simulink library "eng_simple_transient_std"  (Simulink 8.7)
settings: Solver=ode45  StartTime=0.0  StopTime=10.0  RelTol=1e-3
undefined symbols (not defined in the file): DiscIntNeverNeededParam, sMP
libraries: simulink x17
(part 2 of 3)

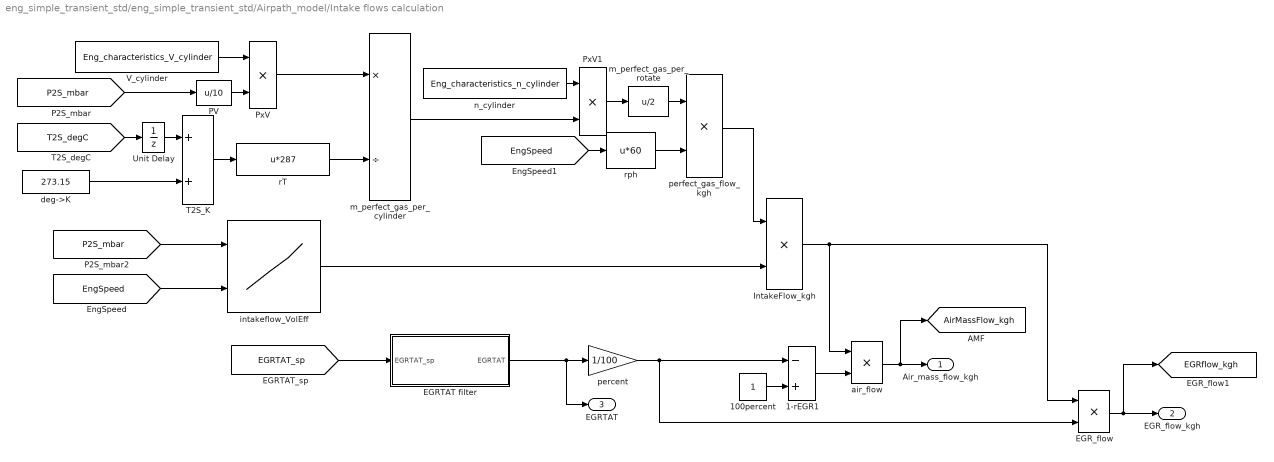
== system eng_simple_transient_std/eng_simple_transient_std/Airpath_model/Intake flows calculation ==
  1-rEGR1 : Sum  Inputs=-+
  100percent : Constant
  EGRTAT filter : Subsystem  AncestorBlock=ControlLib/# First order filter
  EGR_flow : Product  Inputs=**
  IntakeFlow_kgh : Product  RndMeth=Zero
  PV : Fcn  Expr=u/10
  PxV : Product  RndMeth=Zero
  PxV1 : Product  RndMeth=Zero
  T2S_K : Sum
  Unit Delay : UnitDelay  SampleTime=-1
  V_cylinder : Constant  Value=Eng_characteristics_V_cylinder
  air_flow : Product  Inputs=**
  deg->K : Constant  Value=273.15
  intakeflow_VolEff : Lookup2D  RowIndex=Airpath_intakeflow_y_P2S_mbar  ColumnIndex=Airpath_intakeflow_x_NMOTW_rpm  Table=Airpath_intakeflow_z_VolEff  LookUpMeth=Interpolation-Use End Values
  m_perfect_gas_per_cylinder : Product  Inputs=*/
  m_perfect_gas_per_rotate : Fcn  Expr=u/2
  n_cylinder : Constant  Value=Eng_characteristics_n_cylinder
  percent : Gain  Gain=1/100
  perfect_gas_flow_kgh : Product  RndMeth=Zero
  rT : Fcn  Expr=u*287
  rph : Fcn  Expr=u*60
  Air_mass_flow_kgh : Outport
  EGR_flow_kgh : Outport  Port=2
  EGRTAT : Outport  Port=3
  tag scope: AirMassFlow_kgh=global, EGRflow_kgh=global
  wires:
  PxV1/1 -> m_perfect_gas_per_rotate/1
  m_perfect_gas_per_cylinder/1 -> PxV1/2
  n_cylinder/1 -> PxV1/1
  PxV/1 -> m_perfect_gas_per_cylinder/1
  V_cylinder/1 -> PxV/1
  PV/1 -> PxV/2
  Unit Delay/1 -> T2S_K/1
  perfect_gas_flow_kgh/1 -> IntakeFlow_kgh/1
  rph/1 -> perfect_gas_flow_kgh/2
  m_perfect_gas_per_rotate/1 -> perfect_gas_flow_kgh/1
  [EngSpeed] -> rph/1
  [P2S_mbar] -> intakeflow_VolEff/1
  [EngSpeed] -> intakeflow_VolEff/2
  [P2S_mbar] -> PV/1
  deg->K/1 -> T2S_K/2
  [T2S_degC] -> Unit Delay/1
  rT/1 -> m_perfect_gas_per_cylinder/2
  T2S_K/1 -> rT/1
  intakeflow_VolEff/1 -> IntakeFlow_kgh/2
  IntakeFlow_kgh/1 -> air_flow/1, EGR_flow/1
  [EGRTAT_sp] -> EGRTAT filter/1(EGRTAT_sp)
  EGRTAT filter/1(EGRTAT) -> EGRTAT/1, percent/1
  100percent/1 -> 1-rEGR1/2
  percent/1 -> EGR_flow/2, 1-rEGR1/1
  1-rEGR1/1 -> air_flow/2
  EGR_flow/1 -> [EGRflow_kgh], EGR_flow_kgh/1
  air_flow/1 -> [AirMassFlow_kgh], Air_mass_flow_kgh/1

== system eng_simple_transient_std/eng_simple_transient_std/Engine_model/AFR calculation ==
  AFR calc : Product  Inputs=*//
  Saturation : Saturate  UpperLimit=20  LowerLimit=0
  Saturation1 : Saturate  UpperLimit=1e6  LowerLimit=1e-6
  Stoech_coeff : Constant  Value=Eng_characteristics_Stoech_coeff
  AFR : Outport
  wires:
  [MFuel_kgh] -> Saturation1/1
  Saturation1/1 -> AFR calc/2
  Saturation/1 -> AFR/1
  AFR calc/1 -> Saturation/1
  Stoech_coeff/1 -> AFR calc/3
  [AirMassFlow_kgh] -> AFR calc/1

== system eng_simple_transient_std/eng_simple_transient_std/Engine_model/AdBlue consumption ==
  Calc_AdBlue_Consumption : Subsystem
  Discrete-Time Integrator : DiscreteIntegrator  SampleTime=-1  ICPrevOutput=DiscIntNeverNeededParam  ICPrevScaledInput=DiscIntNeverNeededParam
  Divide : Product  Inputs=*/
  Divide1 : Product  Inputs=*/
  fuel_density : Constant  Value=Eng_characteristics_AdBlue_density
  kgh->kgs : Gain  Gain=1/3600
  MAdBlue_brk_kgh : Outport
  VAdBlue_Lh : Outport  Port=2
  MAdBlue_kg : Outport  Port=3
  VAdBlue_L : Outport  Port=4
  wires:
  Calc_AdBlue_Consumption/1(MAdBlue_brk_kgh) -> Divide/1, kgh->kgs/1, MAdBlue_brk_kgh/1
  [MAdBlue_kgh] -> Calc_AdBlue_Consumption/2(MAdBlue_kgh)
  Divide/1 -> VAdBlue_Lh/1
  fuel_density/1 -> Divide/2, Divide1/2
  Divide1/1 -> VAdBlue_L/1
  kgh->kgs/1 -> Discrete-Time Integrator/1
  [brakingMode] -> Calc_AdBlue_Consumption/1(brakingMode)
  Discrete-Time Integrator/1 -> MAdBlue_kg/1, Divide1/1

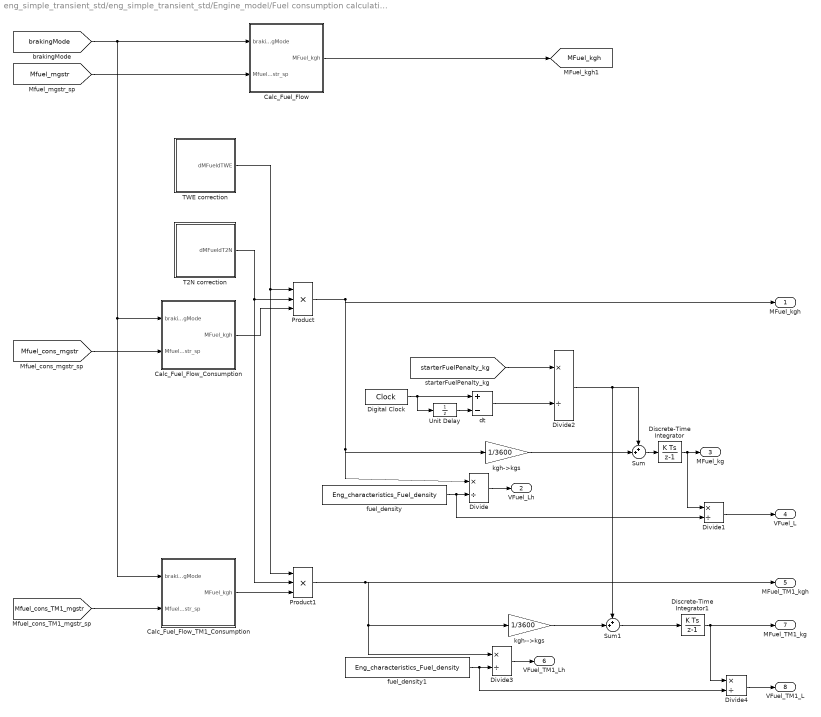
== system eng_simple_transient_std/eng_simple_transient_std/Engine_model/Fuel consumption calculation ==
  Calc_Fuel_Flow : Subsystem
  Calc_Fuel_Flow_Consumption : Subsystem
  Calc_Fuel_Flow_TM1_Consumption : Subsystem
  Digital Clock : DigitalClock  SampleTime=-1
  Discrete-Time Integrator : DiscreteIntegrator  SampleTime=-1  ICPrevOutput=DiscIntNeverNeededParam  ICPrevScaledInput=DiscIntNeverNeededParam
  Discrete-Time Integrator1 : DiscreteIntegrator  SampleTime=-1  ICPrevOutput=DiscIntNeverNeededParam  ICPrevScaledInput=DiscIntNeverNeededParam
  Divide{,1..4} (5 alike) : Product  Inputs=*/
  Product : Product  Inputs=3  RndMeth=Zero
  Product1 : Product  Inputs=3  RndMeth=Zero
  Sum : Sum  Inputs=++|
  Sum1 : Sum  Inputs=++|
  T2N correction : Subsystem
  TWE correction : Subsystem
  Unit Delay : UnitDelay  InitialCondition=-1  SampleTime=-1
  dt : Sum  Inputs=+-
  fuel_density : Constant  Value=Eng_characteristics_Fuel_density
  fuel_density1 : Constant  Value=Eng_characteristics_Fuel_density
  kgh-->kgs : Gain  Gain=1/3600
  kgh->kgs : Gain  Gain=1/3600
  MFuel_kgh : Outport
  VFuel_Lh : Outport  Port=2
  MFuel_kg : Outport  Port=3
  VFuel_L : Outport  Port=4
  MFuel_TM1_kgh : Outport  Port=5
  VFuel_TM1_Lh : Outport  Port=6
  MFuel_TM1_kg : Outport  Port=7
  VFuel_TM1_L : Outport  Port=8
  tag scope: MFuel_kgh=global
  wires:
  Divide2/1 -> Sum/1, Sum1/1
  dt/1 -> Divide2/2
  [starterFuelPenalty_kg] -> Divide2/1
  Digital Clock/1 -> dt/1, Unit Delay/1
  Unit Delay/1 -> dt/2
  Discrete-Time Integrator/1 -> Divide1/1, MFuel_kg/1
  Sum/1 -> Discrete-Time Integrator/1
  Calc_Fuel_Flow/1(MFuel_kgh) -> [MFuel_kgh]
  [brakingMode] -> Calc_Fuel_Flow/1(brakingMode), Calc_Fuel_Flow_Consumption/1(brakingMode), Calc_Fuel_Flow_TM1_Consumption/1(brakingMode)
  kgh->kgs/1 -> Sum/2
  Divide1/1 -> VFuel_L/1
  fuel_density/1 -> Divide1/2, Divide/2
  Divide/1 -> VFuel_Lh/1
  [Mfuel_mgstr] -> Calc_Fuel_Flow/2(Mfuel_mgstr_sp)
  [Mfuel_cons_mgstr] -> Calc_Fuel_Flow_Consumption/2(Mfuel_mgstr_sp)
  T2N correction/1(dMFueldT2N) -> Product/2, Product1/2
  Product/1 -> MFuel_kgh/1, kgh->kgs/1, Divide/1
  [Mfuel_cons_TM1_mgstr] -> Calc_Fuel_Flow_TM1_Consumption/2(Mfuel_mgstr_sp)
  Product1/1 -> MFuel_TM1_kgh/1, Divide3/1, kgh-->kgs/1
  Discrete-Time Integrator1/1 -> Divide4/1, MFuel_TM1_kg/1
  Sum1/1 -> Discrete-Time Integrator1/1
  kgh-->kgs/1 -> Sum1/2
  Divide4/1 -> VFuel_TM1_L/1
  fuel_density1/1 -> Divide4/2, Divide3/2
  Divide3/1 -> VFuel_TM1_Lh/1
  Calc_Fuel_Flow_Consumption/1(MFuel_kgh) -> Product/3
  TWE correction/1(dMFueldTWE) -> Product/1, Product1/1
  Calc_Fuel_Flow_TM1_Consumption/1(MFuel_kgh) -> Product1/3

== system eng_simple_transient_std/eng_simple_transient_std/Engine_model/cooler_model ==
  Abs : Abs
  Compare To Zero : simulink/Logic and Bit Operations/Compare To Zero  relop=<=  OutDataTypeStr=uint8
  Constant : Constant  Value=Thermal_heatRelease_negTorque_factor
  Constant1 : Constant
  Heatrelease_kW : Lookup2D  RowIndex=Thermal_heatRelease_y_Torque_Nm  ColumnIndex=Thermal_heatRelease_x_NMOT_rpm  Table=Thermal_heatRelease_z_heat_kW
  Product : Product  RndMeth=Zero
  Switch : Switch  Criteria=u2 > Threshold
  eng_HeatMean_power : Outport
  wires:
  [EngSpeed] -> Heatrelease_kW/2
  [Torque_Nm_sp] -> Compare To Zero/1, Abs/1
  Compare To Zero/1 -> Switch/2
  Constant/1 -> Switch/1
  Constant1/1 -> Switch/3
  Heatrelease_kW/1 -> Product/2  "eng_HeatMean_power_raw"
  Product/1 -> eng_HeatMean_power/1  "eng_HeatMean_power"
  Switch/1 -> Product/1
  Abs/1 -> Heatrelease_kW/1

== system eng_simple_transient_std/eng_simple_transient_std/Outputs/Calc_exhGas ==
  AFR : Inport
  haluft for Ttau 10°C praum 1013mbar : Constant  Value=7.56
  rCO2_calc : Subsystem
  rH2O_calc : Subsystem  AncestorBlock=|
      | ExACT_Custom_Tools/direct input/Wasser Raumanteil Abgas
      | rH2O_Abg[-] = f(lambda[-],TTau[°C],pambL[mbar])
  rO2_calc : Subsystem  AncestorBlock=|
      | ExACT_Custom_Tools/direct input/Sauerstoff Raumanteil Abgas
      | rO2_Abg[-] = f(lambda[-],TTau[°C],pambL[mbar])
  rCO2_Abg : Outport
  rH2O_Abg : Outport  Port=2
  rO2_Abg : Outport  Port=3
  wires:
  rCO2_calc/1(CO2_molfrac) -> rCO2_Abg/1
  AFR/1 -> rCO2_calc/1(AFR), rO2_calc/1(AFR), rH2O_calc/1(AFR)
  haluft for Ttau 10°C praum 1013mbar/1 -> rCO2_calc/2(haluft), rO2_calc/2(haluft), rH2O_calc/2(haluft)
  rH2O_calc/1(rH2O_Abg) -> rH2O_Abg/1
  rO2_calc/1(rO2_Abg) -> rO2_Abg/1

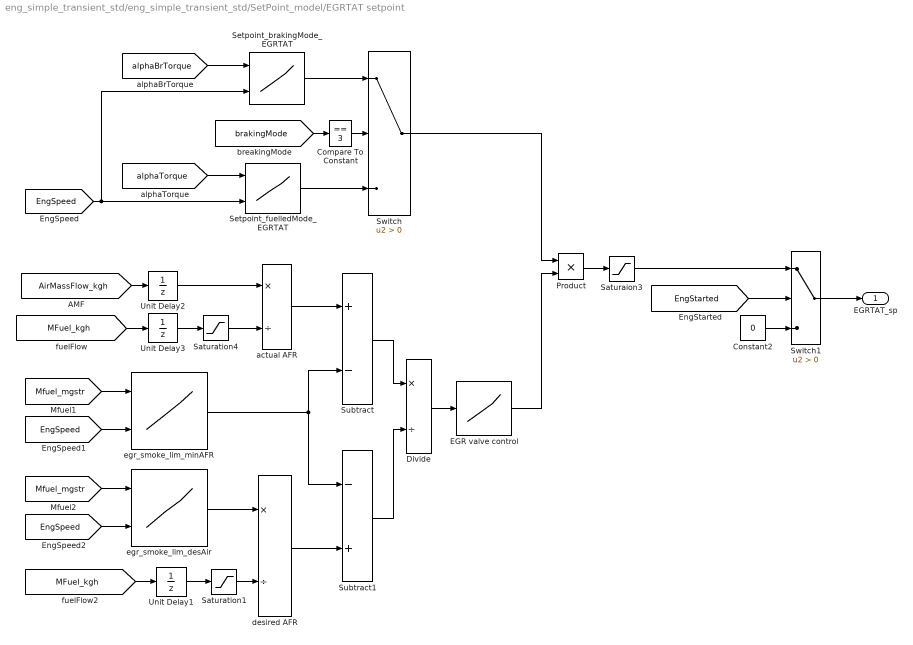
== system eng_simple_transient_std/eng_simple_transient_std/SetPoint_model/EGRTAT setpoint ==
  Compare To Constant : simulink/Logic and Bit Operations/Compare To Constant  relop===  const=3  OutDataTypeStr=uint8
      link override Compare: Operator===
  Constant2 : Constant  Value=0
  Divide : Product  Inputs=*/
  EGR valve control : Lookup  InputValues=Fiter_calibration_fmode_y_ec_EGRTAT  Table=[0 1]  LookUpMeth=Interpolation-Use End Values
  Product : Product  RndMeth=Zero
  Saturaion3 : Saturate  UpperLimit=100  LowerLimit=0
  Saturation1 : Saturate  UpperLimit=1e6  LowerLimit=1e-6
  Saturation4 : Saturate  UpperLimit=1e6  LowerLimit=1e-6
  Setpoint_brakingMode_EGRTAT : Lookup2D  RowIndex=Setpoint_brakingMode3_y_alphaTorque  ColumnIndex=Setpoint_brakingMode3_x_NMOTW_rpm  Table=Setpoint_brakingMode3_z_EGRTAT
  Setpoint_fuelledMode_EGRTAT : Lookup2D  RowIndex=Setpoint_fuelledMode_y_alphaTorque  ColumnIndex=Setpoint_fuelledMode_x_NMOTW_rpm  Table=Setpoint_fuelledMode_z_EGRTAT
  Subtract : Sum  Inputs=+-
  Subtract1 : Sum  Inputs=-+
  Switch : Switch  Criteria=u2 > Threshold
  Switch1 : Switch  Criteria=u2 > Threshold
  Unit Delay1 : UnitDelay  SampleTime=-1
  Unit Delay2 : UnitDelay  SampleTime=-1
  Unit Delay3 : UnitDelay  SampleTime=-1
  actual AFR : Product  Inputs=*/
  desired AFR : Product  Inputs=*/
  egr_smoke_lim_desAir : Lookup2D  Description=|  RowIndex=egr_smoke_lim_y_Mfuel_mgstr  ColumnIndex=egr_smoke_lim_x_NMOT_rpm  Table=egr_smoke_lim_z_desAir_kgh  LookUpMeth=Interpolation-Use End Values  OutDataTypeStr=double
      | Look-up table (2D) of dSPACE TargetLink.
      | 
      | This block calculates the output values dependant on the given table matrix. Note that both the row and column index vectors must be monotonically increasing for TargetLink.
  egr_smoke_lim_minAFR : Lookup2D  Description=|  RowIndex=egr_smoke_lim_y_Mfuel_mgstr  ColumnIndex=egr_smoke_lim_x_NMOT_rpm  Table=egr_smoke_lim_z_minAFR  LookUpMeth=Interpolation-Use End Values  OutDataTypeStr=double
      | Look-up table (2D) of dSPACE TargetLink.
      | 
      | This block calculates the output values dependant on the given table matrix. Note that both the row and column index vectors must be monotonically increasing for TargetLink.
  EGRTAT_sp : Outport
  wires:
  Setpoint_fuelledMode_EGRTAT/1 -> Switch/3
  Setpoint_brakingMode_EGRTAT/1 -> Switch/1
  [EngSpeed] -> Setpoint_brakingMode_EGRTAT/2, Setpoint_fuelledMode_EGRTAT/2
  [brakingMode] -> Compare To Constant/1
  Switch1/1 -> EGRTAT_sp/1
  Saturaion3/1 -> Switch1/1
  Constant2/1 -> Switch1/3
  [EngStarted] -> Switch1/2
  EGR valve control/1 -> Product/2
  Divide/1 -> EGR valve control/1
  Subtract1/1 -> Divide/2
  Subtract/1 -> Divide/1
  desired AFR/1 -> Subtract1/2
  actual AFR/1 -> Subtract/1
  egr_smoke_lim_desAir/1 -> desired AFR/1
  Saturation1/1 -> desired AFR/2
  Unit Delay1/1 -> Saturation1/1
  [MFuel_kgh] -> Unit Delay1/1
  [EngSpeed] -> egr_smoke_lim_desAir/2
  [Mfuel_mgstr] -> egr_smoke_lim_desAir/1
  egr_smoke_lim_minAFR/1 -> Subtract1/1, Subtract/2
  Saturation4/1 -> actual AFR/2
  Unit Delay3/1 -> Saturation4/1
  Unit Delay2/1 -> actual AFR/1
  [MFuel_kgh] -> Unit Delay3/1
  [AirMassFlow_kgh] -> Unit Delay2/1
  [EngSpeed] -> egr_smoke_lim_minAFR/2
  [Mfuel_mgstr] -> egr_smoke_lim_minAFR/1
  Product/1 -> Saturaion3/1
  Switch/1 -> Product/1
  [alphaBrTorque] -> Setpoint_brakingMode_EGRTAT/1
  [alphaTorque] -> Setpoint_fuelledMode_EGRTAT/1
  Compare To Constant/1 -> Switch/2

== system eng_simple_transient_std/eng_simple_transient_std/SetPoint_model/Mass of fuel injected TM1 ==
  mcm_wfa_wf_smoke : Inport
  Constant2 : Constant
  Product : Product  RndMeth=Zero
  Product1 : Product  RndMeth=Zero
  Saturation1 : Saturate  UpperLimit=1e6  LowerLimit=-1
  Saturation2 : Saturate  UpperLimit=1e6  LowerLimit=0
  Saturation3 : Saturate  UpperLimit=1  LowerLimit=0
  Setpoint_fuelledMode_Smoke : Lookup2D  RowIndex=Setpoint_fuelledMode_y_alphaTorque  ColumnIndex=Setpoint_fuelledMode_x_NMOTW_rpm  Table=Setpoint_fuelledMode_z_Mfuel_smoke_factor
  Setpoint_fuelledMode_TM1_Mfuel : Lookup2D  RowIndex=Setpoint_fuelledMode_y_alphaTorque  ColumnIndex=Setpoint_fuelledMode_x_NMOTW_rpm  Table=Setpoint_fuelledMode_z_Mfuel_TM1_mgstr
  Sum1 : Sum  Inputs=|++
  Mfuel_consumption_TM1_mgstr : Outport
  wires:
  Product1/1 -> Mfuel_consumption_TM1_mgstr/1
  Saturation2/1 -> Product1/1
  Sum1/1 -> Product1/2
  Product/1 -> Sum1/2
  Constant2/1 -> Sum1/1
  Saturation3/1 -> Product/2
  Saturation1/1 -> Product/1
  mcm_wfa_wf_smoke/1 -> Saturation3/1
  Setpoint_fuelledMode_Smoke/1 -> Saturation1/1
  [alphaTorque] -> Setpoint_fuelledMode_Smoke/1, Setpoint_fuelledMode_TM1_Mfuel/1
  [EngSpeed] -> Setpoint_fuelledMode_Smoke/2, Setpoint_fuelledMode_TM1_Mfuel/2
  Setpoint_fuelledMode_TM1_Mfuel/1 -> Saturation2/1

== system eng_simple_transient_std/eng_simple_transient_std/SetPoint_model/Mass of fuel injected setpoint ==
  mcm_fbf_des_fuel_mass : Inport
  mcm_wfa_wf_smoke : Inport  Port=2
  Constant : Constant  Value=Eng_characteristics_Mfuel_available
  Constant1 : Constant  Value=Eng_characteristics_Mfuel_with_MCM
  Constant2 : Constant
  Product : Product  RndMeth=Zero
  Product1 : Product  RndMeth=Zero
  Saturation1 : Saturate  UpperLimit=1e6  LowerLimit=-1
  Saturation2 : Saturate  UpperLimit=1e6  LowerLimit=0
  Saturation3 : Saturate  UpperLimit=1  LowerLimit=0
  Setpoint_fuelledMode_Mfuel : Lookup2D  RowIndex=Setpoint_fuelledMode_y_alphaTorque  ColumnIndex=Setpoint_fuelledMode_x_NMOTW_rpm  Table=Setpoint_fuelledMode_z_Mfuel_mgstr
  Setpoint_fuelledMode_Smoke : Lookup2D  RowIndex=Setpoint_fuelledMode_y_alphaTorque  ColumnIndex=Setpoint_fuelledMode_x_NMOTW_rpm  Table=Setpoint_fuelledMode_z_Mfuel_smoke_factor
  Sum1 : Sum  Inputs=|++
  Switch : Switch  Criteria=u2 > Threshold
  Switch1 : Switch  Criteria=u2 > Threshold
  Mfuel_mgstr : Outport
  Mfuel_consumption_mgstr : Outport  Port=2
  wires:
  Switch/1 -> Mfuel_mgstr/1
  mcm_fbf_des_fuel_mass/1 -> Switch/1, Switch1/1
  Constant/1 -> Switch/2
  Setpoint_fuelledMode_Mfuel/1 -> Saturation2/1
  [EngSpeed] -> Setpoint_fuelledMode_Mfuel/2, Setpoint_fuelledMode_Smoke/2
  [alphaTorque] -> Setpoint_fuelledMode_Mfuel/1, Setpoint_fuelledMode_Smoke/1
  Constant1/1 -> Switch1/2
  Switch1/1 -> Mfuel_consumption_mgstr/1
  Setpoint_fuelledMode_Smoke/1 -> Saturation1/1
  mcm_wfa_wf_smoke/1 -> Saturation3/1
  Saturation1/1 -> Product/1
  Saturation3/1 -> Product/2
  Constant2/1 -> Sum1/1
  Product/1 -> Sum1/2
  Sum1/1 -> Product1/2
  Saturation2/1 -> Product1/1
  Product1/1 -> Switch/3, Switch1/3

== system eng_simple_transient_std/eng_simple_transient_std/SetPoint_model/P2S setpoint ==
  Gain : Gain  Gain=1/2
  Gain1 : Gain  Gain=1/2
  Multiport Switch2 : MultiPortSwitch  DataPortOrder=Zero-based contiguous  Inputs=5  zeroidx=on
  Setpoint_Friction_P2S : Lookup2D  RowIndex=Setpoint_fuelledMode_y_alphaTorque  ColumnIndex=Setpoint_fuelledMode_x_NMOTW_rpm  Table=Setpoint_fuelledMode_z_P2S_mbar
  Setpoint_brakingMode1_P2S : Lookup2D  RowIndex=Setpoint_brakingMode1_y_alphaTorque  ColumnIndex=Setpoint_brakingMode1_x_NMOTW_rpm  Table=Setpoint_brakingMode1_z_P2S_mbar
  Setpoint_brakingMode2_P2S : Lookup2D  RowIndex=Setpoint_brakingMode2_y_alphaTorque  ColumnIndex=Setpoint_brakingMode2_x_NMOTW_rpm  Table=Setpoint_brakingMode2_z_P2S_mbar
  Setpoint_brakingMode3_P2S : Lookup2D  RowIndex=Setpoint_brakingMode3_y_alphaTorque  ColumnIndex=Setpoint_brakingMode3_x_NMOTW_rpm  Table=Setpoint_brakingMode3_z_P2S_mbar
  Setpoint_fuelledMode_P2S : Lookup2D  RowIndex=Setpoint_fuelledMode_y_alphaTorque  ColumnIndex=Setpoint_fuelledMode_x_NMOTW_rpm  Table=Setpoint_fuelledMode_z_P2S_mbar
  Sum1 : Sum  Inputs=|-+
  Sum2 : Sum  Inputs=++|
  Sum3 : Sum  Inputs=++|
  Sum4 : Sum  Inputs=++|
  Switch1 : Switch  Criteria=u2 > Threshold
  alpaTorqueFriction : Constant  Value=0
  P2S_mbar_sp : Outport
  wires:
  Gain/1 -> Sum3/1, Sum2/1
  Sum1/1 -> Gain/1
  Setpoint_Friction_P2S/1 -> Sum1/1, Sum4/2
  alpaTorqueFriction/1 -> Setpoint_Friction_P2S/1
  Multiport Switch2/1 -> Switch1/1
  [env_AirPress] -> Switch1/3
  Switch1/1 -> P2S_mbar_sp/1
  [EngStarted] -> Switch1/2
  Sum3/1 -> Multiport Switch2/4
  Sum2/1 -> Multiport Switch2/3
  Setpoint_brakingMode1_P2S/1 -> Sum2/2
  Setpoint_brakingMode2_P2S/1 -> Sum3/2
  [EngSpeed] -> Setpoint_Friction_P2S/2, Setpoint_fuelledMode_P2S/2, Setpoint_brakingMode1_P2S/2, Setpoint_brakingMode3_P2S/2, Setpoint_brakingMode2_P2S/2
  [alphaTorque] -> Setpoint_fuelledMode_P2S/1
  [alphaBrTorque] -> Setpoint_brakingMode1_P2S/1, Setpoint_brakingMode2_P2S/1, Setpoint_brakingMode3_P2S/1
  Setpoint_fuelledMode_P2S/1 -> Sum1/2, Multiport Switch2/2, Sum4/1
  Setpoint_brakingMode3_P2S/1 -> Multiport Switch2/5
  [brakingMode] -> Multiport Switch2/1
  Sum4/1 -> Gain1/1
  Gain1/1 -> Multiport Switch2/6

== system eng_simple_transient_std/eng_simple_transient_std/SetPoint_model/P31 setpoint ==
  Multiport Switch4 : MultiPortSwitch  DataPortOrder=Zero-based contiguous  Inputs=5  zeroidx=on
  Setpoint_brakingMode1_P31 : Lookup2D  RowIndex=Setpoint_brakingMode1_y_alphaTorque  ColumnIndex=Setpoint_brakingMode1_x_NMOTW_rpm  Table=Setpoint_brakingMode1_z_P31_mbar
  Setpoint_brakingMode3_P31 : Lookup2D  RowIndex=Setpoint_brakingMode3_y_alphaTorque  ColumnIndex=Setpoint_brakingMode3_x_NMOTW_rpm  Table=Setpoint_brakingMode3_z_P31_mbar
  Setpoint_fuelledMode_P31 : Lookup2D  RowIndex=Setpoint_fuelledMode_y_alphaTorque  ColumnIndex=Setpoint_fuelledMode_x_NMOTW_rpm  Table=Setpoint_fuelledMode_z_P31_mbar
  Switch1 : Switch  Criteria=u2 > Threshold
  P31_mbar_sp : Outport
  wires:
  Setpoint_brakingMode1_P31/1 -> Multiport Switch4/3
  Multiport Switch4/1 -> Switch1/1
  [env_AirPress] -> Switch1/3
  Switch1/1 -> P31_mbar_sp/1
  [EngStarted] -> Switch1/2
  [EngSpeed] -> Setpoint_brakingMode3_P31/2, Setpoint_brakingMode1_P31/2, Setpoint_fuelledMode_P31/2
  Setpoint_brakingMode3_P31/1 -> Multiport Switch4/5
  [alphaBrTorque] -> Setpoint_brakingMode1_P31/1, Setpoint_brakingMode3_P31/1
  [alphaTorque] -> Setpoint_fuelledMode_P31/1
  Setpoint_fuelledMode_P31/1 -> Multiport Switch4/2, Multiport Switch4/4, Multiport Switch4/6
  [brakingMode] -> Multiport Switch4/1

== system eng_simple_transient_std/eng_simple_transient_std/SetPoint_model/P32 setpoint ==
  Constant : Constant  Value=0
  Multiport Switch6 : MultiPortSwitch  DataPortOrder=Zero-based contiguous  Inputs=5  zeroidx=on
  Setpoint_brakingMode2_P32 : Lookup2D  RowIndex=Setpoint_brakingMode2_y_alphaTorque  ColumnIndex=Setpoint_brakingMode2_x_NMOTW_rpm  Table=Setpoint_brakingMode2_z_P32_mbar
  Setpoint_brakingMode3_P32 : Lookup2D  RowIndex=Setpoint_brakingMode3_y_alphaTorque  ColumnIndex=Setpoint_brakingMode3_x_NMOTW_rpm  Table=Setpoint_brakingMode3_z_P32_mbar
  Setpoint_fuelledMode_P32 : Lookup2D  RowIndex=Setpoint_fuelledMode_y_alphaTorque  ColumnIndex=Setpoint_fuelledMode_x_NMOTW_rpm  Table=Setpoint_fuelledMode_z_P32_mbar
  Setpoint_fuelledMode_P32_2 : Lookup2D  RowIndex=Setpoint_fuelledMode_y_alphaTorque  ColumnIndex=Setpoint_fuelledMode_x_NMOTW_rpm  Table=Setpoint_fuelledMode_z_P32_mbar
  Switch1 : Switch  Criteria=u2 > Threshold
  P32_mbar_sp : Outport
  wires:
  Setpoint_brakingMode2_P32/1 -> Multiport Switch6/4
  Multiport Switch6/1 -> Switch1/1
  [env_AirPress] -> Switch1/3
  Switch1/1 -> P32_mbar_sp/1
  [EngStarted] -> Switch1/2
  [EngSpeed] -> Setpoint_fuelledMode_P32/2, Setpoint_brakingMode2_P32/2, Setpoint_brakingMode3_P32/2, Setpoint_fuelledMode_P32_2/2
  Setpoint_brakingMode3_P32/1 -> Multiport Switch6/5
  [alphaBrTorque] -> Setpoint_brakingMode2_P32/1, Setpoint_brakingMode3_P32/1
  [alphaTorque] -> Setpoint_fuelledMode_P32/1
  Setpoint_fuelledMode_P32/1 -> Multiport Switch6/3, Multiport Switch6/2
  [brakingMode] -> Multiport Switch6/1
  Constant/1 -> Setpoint_fuelledMode_P32_2/1
  Setpoint_fuelledMode_P32_2/1 -> Multiport Switch6/6

== system eng_simple_transient_std/eng_simple_transient_std/SetPoint_model/Starter model ==
  mcm_b_ignition : Inport
  scl_starter : Inport  Port=2
  Compare To Zero : simulink/Logic and Bit Operations/Compare To Zero  relop===  OutDataTypeStr=uint8
      link override Compare: Operator===
  Data Type Conversion2 : DataTypeConversion  OutDataTypeStr=double
  Detect Decrease1 : simulink/Logic and Bit Operations/Detect Decrease  vinit=0  InputProcessing=Inherited  OutDataTypeStr=uint8
  Detect Decrease2 : simulink/Logic and Bit Operations/Detect Decrease  vinit=0  InputProcessing=Inherited  OutDataTypeStr=uint8
  Detect Decrease4 : simulink/Logic and Bit Operations/Detect Decrease  vinit=0  InputProcessing=Inherited  OutDataTypeStr=uint8
  Detect Increase : simulink/Logic and Bit Operations/Detect Increase  vinit=0.0  InputProcessing=Inherited  OutDataTypeStr=uint8
  Eng_starter_fuel_penalty_kg : Constant  Value=Eng_starter_fuel_penalty_kg
  Product : Product  RndMeth=Zero
  Starter engaged : Logic  Inputs=3  AllPortsSameDT=off  OutDataTypeStr=boolean
  Starter_initialisation : Step  Time=0.1  Before=Eng_initialisation_eng_started  After=0
  Status change : Logic  Operator=OR  Inputs=3  AllPortsSameDT=off  OutDataTypeStr=boolean
  Switch1 : Switch  Criteria=u2 > Threshold
  Unit Delay4 : UnitDelay  SampleTime=-1
  b_ignition1 : InportShadow
  engStarted actualisation : Subsystem  TreatAsAtomicUnit=on
  starter torque : Constant  Value=Eng_starter_torque_Nm
  starter torque filter : Subsystem  AncestorBlock=ControlLib/# First order filter
  zero torque : Constant  Value=0
  EngStarted : Outport
  tag scope: starterFuelPenalty_kg=global, starterTorque=global
  wires:
  Eng_starter_fuel_penalty_kg/1 -> Product/1
  Product/1 -> [starterFuelPenalty_kg]
  Detect Decrease2/1 -> Status change/3
  Data Type Conversion2/1 -> Product/2
  Starter_initialisation/1 -> Detect Decrease2/1
  Detect Increase/1 -> Data Type Conversion2/1
  b_ignition1/1 -> engStarted actualisation/1(b_ignition)
  engStarted actualisation/1(EngStarted) -> Unit Delay4/1
  Status change/1 -> engStarted actualisation/Trigger
  Compare To Zero/1 -> Starter engaged/1
  mcm_b_ignition/1 -> Detect Decrease1/1, Starter engaged/3
  Detect Decrease1/1 -> Status change/2
  Detect Decrease4/1 -> Status change/1
  [EngStarted] -> Compare To Zero/1
  starter torque filter/1(starterTorque) -> [starterTorque]
  starter torque/1 -> Switch1/1
  Starter engaged/1 -> Detect Increase/1, Detect Decrease4/1, Switch1/2
  scl_starter/1 -> Starter engaged/2
  Unit Delay4/1 -> EngStarted/1
  Switch1/1 -> starter torque filter/1(starterTorque_sp)
  zero torque/1 -> Switch1/3

== system eng_simple_transient_std/eng_simple_transient_std/SetPoint_model/T2N setpoint ==
  Setpoint_fuelledMode_T2N : Lookup2D  RowIndex=Setpoint_fuelledMode_y_alphaTorque  ColumnIndex=Setpoint_fuelledMode_x_NMOTW_rpm  Table=Setpoint_fuelledMode_z_T2N_degC
  Switch1 : Switch  Criteria=u2 > Threshold
  T2N_degC_sp : Outport
  wires:
  [env_AirTemp] -> Switch1/3
  Switch1/1 -> T2N_degC_sp/1
  [EngStarted] -> Switch1/2
  [alphaTorque] -> Setpoint_fuelledMode_T2N/1
  Setpoint_fuelledMode_T2N/1 -> Switch1/1
  [EngSpeed] -> Setpoint_fuelledMode_T2N/2

== system eng_simple_transient_std/eng_simple_transient_std/SetPoint_model/T31 setpoint ==
  Multiport Switch5 : MultiPortSwitch  DataPortOrder=Zero-based contiguous  Inputs=5  zeroidx=on
  Setpoint_brakingMode1_T31 : Lookup2D  RowIndex=Setpoint_brakingMode1_y_alphaTorque  ColumnIndex=Setpoint_brakingMode1_x_NMOTW_rpm  Table=Setpoint_brakingMode1_z_T31_degC
  Setpoint_brakingMode3_T31 : Lookup2D  RowIndex=Setpoint_brakingMode3_y_alphaTorque  ColumnIndex=Setpoint_brakingMode3_x_NMOTW_rpm  Table=Setpoint_brakingMode3_z_T31_degC
  Setpoint_fuelledMode_T31 : Lookup2D  RowIndex=Setpoint_fuelledMode_y_alphaTorque  ColumnIndex=Setpoint_fuelledMode_x_NMOTW_rpm  Table=Setpoint_fuelledMode_z_T31_degC
  Switch1 : Switch  Criteria=u2 > Threshold
  T31_degC_sp : Outport
  wires:
  Setpoint_brakingMode1_T31/1 -> Multiport Switch5/3
  Multiport Switch5/1 -> Switch1/1
  [eng_CoolantEngineOut_Temperature] -> Switch1/3
  Switch1/1 -> T31_degC_sp/1
  [EngStarted] -> Switch1/2
  [alphaBrTorque] -> Setpoint_brakingMode1_T31/1, Setpoint_brakingMode3_T31/1
  [alphaTorque] -> Setpoint_fuelledMode_T31/1
  [EngSpeed] -> Setpoint_brakingMode1_T31/2, Setpoint_brakingMode3_T31/2, Setpoint_fuelledMode_T31/2
  Setpoint_fuelledMode_T31/1 -> Multiport Switch5/2, Multiport Switch5/4, Multiport Switch5/6
  Setpoint_brakingMode3_T31/1 -> Multiport Switch5/5
  [brakingMode] -> Multiport Switch5/1

== system eng_simple_transient_std/eng_simple_transient_std/SetPoint_model/T32 setpoint ==
  Constant1 : Constant  Value=0
  Multiport Switch7 : MultiPortSwitch  DataPortOrder=Zero-based contiguous  Inputs=5  zeroidx=on
  Setpoint_brakingMode2_T32 : Lookup2D  RowIndex=Setpoint_brakingMode2_y_alphaTorque  ColumnIndex=Setpoint_brakingMode2_x_NMOTW_rpm  Table=Setpoint_brakingMode2_z_T32_degC
  Setpoint_brakingMode3_T32 : Lookup2D  RowIndex=Setpoint_brakingMode3_y_alphaTorque  ColumnIndex=Setpoint_brakingMode3_x_NMOTW_rpm  Table=Setpoint_brakingMode3_z_T32_degC
  Setpoint_fuelledMode_T32 : Lookup2D  RowIndex=Setpoint_fuelledMode_y_alphaTorque  ColumnIndex=Setpoint_fuelledMode_x_NMOTW_rpm  Table=Setpoint_fuelledMode_z_T32_degC
  Setpoint_fuelledMode_T32_2 : Lookup2D  RowIndex=Setpoint_fuelledMode_y_alphaTorque  ColumnIndex=Setpoint_fuelledMode_x_NMOTW_rpm  Table=Setpoint_fuelledMode_z_T32_degC
  Switch1 : Switch  Criteria=u2 > Threshold
  T32_degC_sp : Outport
  wires:
  Setpoint_brakingMode2_T32/1 -> Multiport Switch7/4
  Multiport Switch7/1 -> Switch1/1
  [eng_CoolantEngineOut_Temperature] -> Switch1/3
  Switch1/1 -> T32_degC_sp/1
  [EngStarted] -> Switch1/2
  [alphaBrTorque] -> Setpoint_brakingMode3_T32/1, Setpoint_brakingMode2_T32/1
  [alphaTorque] -> Setpoint_fuelledMode_T32/1
  [EngSpeed] -> Setpoint_fuelledMode_T32/2, Setpoint_brakingMode2_T32/2, Setpoint_brakingMode3_T32/2, Setpoint_fuelledMode_T32_2/2
  Setpoint_fuelledMode_T32/1 -> Multiport Switch7/3, Multiport Switch7/2
  Setpoint_brakingMode3_T32/1 -> Multiport Switch7/5
  [brakingMode] -> Multiport Switch7/1
  Setpoint_fuelledMode_T32_2/1 -> Multiport Switch7/6
  Constant1/1 -> Setpoint_fuelledMode_T32_2/1

== system eng_simple_transient_std/eng_simple_transient_std/SetPoint_model/TWE setpoint ==
  Setpoint_fuelledMode_TWE : Lookup2D  RowIndex=Setpoint_fuelledMode_y_alphaTorque  ColumnIndex=Setpoint_fuelledMode_x_NMOTW_rpm  Table=Setpoint_fuelledMode_z_TWE_degC
  Switch1 : Switch  Criteria=u2 > Threshold
  TWE_degC_sp : Outport
  wires:
  Setpoint_fuelledMode_TWE/1 -> Switch1/1
  [EngSpeed] -> Setpoint_fuelledMode_TWE/2
  [alphaTorque] -> Setpoint_fuelledMode_TWE/1
  [EngStarted] -> Switch1/2
  Switch1/1 -> TWE_degC_sp/1
  [env_AirTemp] -> Switch1/3

== system eng_simple_transient_std/eng_simple_transient_std/SetPoint_model/Torque setpoint ==
  Alpha_p2s_Br1 calculation : Subsystem
  Alpha_p2s_Br2 calculation : Subsystem
  Alpha_p2s_Br3 calculation : Subsystem
  Gain : Gain  Gain=1/2
  Gain1 : Gain  Gain=1/2
  Multiport Switch : MultiPortSwitch  DataPortOrder=Zero-based contiguous  Inputs=5  zeroidx=on
  Setpoint_brakingMode1_Torque : Lookup2D  RowIndex=Setpoint_brakingMode1_y_alphaTorque  ColumnIndex=Setpoint_brakingMode1_x_NMOTW_rpm  Table=Setpoint_brakingMode1_z_Torque_Nm
  Setpoint_brakingMode2_Torque : Lookup2D  RowIndex=Setpoint_brakingMode2_y_alphaTorque  ColumnIndex=Setpoint_brakingMode2_x_NMOTW_rpm  Table=Setpoint_brakingMode2_z_Torque_Nm
  Setpoint_brakingMode3_Torque : Lookup2D  RowIndex=Setpoint_brakingMode3_y_alphaTorque  ColumnIndex=Setpoint_brakingMode3_x_NMOTW_rpm  Table=Setpoint_brakingMode3_z_Torque_Nm
  Setpoint_friction_Torque : Lookup2D  RowIndex=Setpoint_fuelledMode_y_alphaTorque  ColumnIndex=Setpoint_fuelledMode_x_NMOTW_rpm  Table=Setpoint_fuelledMode_z_Torque_Nm
  Setpoint_fuelledMode_Torque : Lookup2D  RowIndex=Setpoint_fuelledMode_y_alphaTorque  ColumnIndex=Setpoint_fuelledMode_x_NMOTW_rpm  Table=Setpoint_fuelledMode_z_Torque_Nm
  Sum1 : Sum  Inputs=|-+
  Sum2 : Sum  Inputs=++|
  Sum3 : Sum  Inputs=++|
  Sum4 : Sum  Inputs=++|
  Switch1 : Switch  Criteria=u2 > Threshold
  Unit Delay2 : UnitDelay  InitialCondition=1e3  SampleTime=-1
  alpaTorqueFriction : Constant  Value=0
  Torque_Nm_sp : Outport
  wires:
  Alpha_p2s_Br3 calculation/1(alpha_p2s_br3) -> Setpoint_brakingMode3_Torque/1
  Alpha_p2s_Br2 calculation/1(alpha_p2s_br2) -> Setpoint_brakingMode2_Torque/1
  Alpha_p2s_Br1 calculation/1(alpha_p2s_br1) -> Setpoint_brakingMode1_Torque/1
  [P2S_mbar] -> Unit Delay2/1
  Unit Delay2/1 -> Alpha_p2s_Br3 calculation/1(p2s), Alpha_p2s_Br2 calculation/1(p2s), Alpha_p2s_Br1 calculation/1(p2s)
  Gain/1 -> Sum3/1, Sum2/1
  Setpoint_friction_Torque/1 -> Sum1/1, Sum4/2
  Sum1/1 -> Gain/1
  Multiport Switch/1 -> Switch1/1
  [starterTorque] -> Switch1/3
  Switch1/1 -> Torque_Nm_sp/1
  [EngStarted] -> Switch1/2
  alpaTorqueFriction/1 -> Setpoint_friction_Torque/1
  Sum3/1 -> Multiport Switch/4
  Setpoint_brakingMode2_Torque/1 -> Sum3/2
  Setpoint_brakingMode1_Torque/1 -> Sum2/2
  Sum2/1 -> Multiport Switch/3
  Setpoint_fuelledMode_Torque/1 -> Sum1/2, Multiport Switch/2, Sum4/1
  Setpoint_brakingMode3_Torque/1 -> Multiport Switch/5
  [EngSpeed] -> Setpoint_fuelledMode_Torque/2, Alpha_p2s_Br3 calculation/2(EngSpeed), Alpha_p2s_Br2 calculation/2(EngSpeed), Alpha_p2s_Br1 calculation/2(EngSpeed), Setpoint_friction_Torque/2, Setpoint_brakingMode3_Torque/2, Setpoint_brakingMode2_Torque/2, Setpoint_brakingMode1_Torque/2
  [alphaTorque] -> Setpoint_fuelledMode_Torque/1
  [brakingMode] -> Multiport Switch/1
  Sum4/1 -> Gain1/1
  Gain1/1 -> Multiport Switch/6

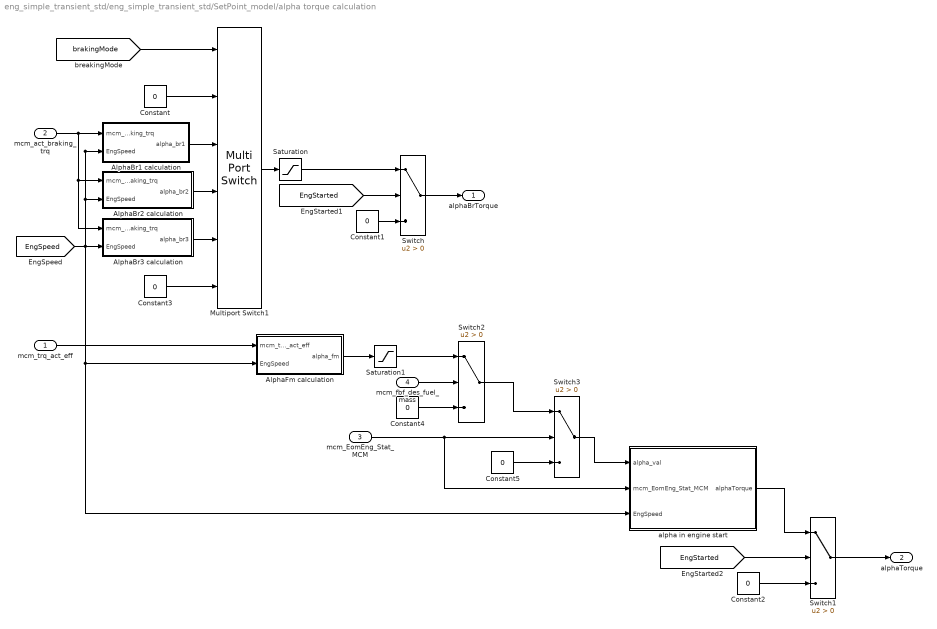
== system eng_simple_transient_std/eng_simple_transient_std/SetPoint_model/alpha torque calculation ==
  mcm_trq_act_eff : Inport
  mcm_act_braking_trq : Inport  Port=2
  mcm_EomEng_Stat_MCM : Inport  Port=3
  mcm_fbf_des_fuel_mass : Inport  Port=4
  AlphaBr1 calculation : Subsystem
  AlphaBr2 calculation : Subsystem
  AlphaBr3 calculation : Subsystem
  AlphaFm calculation : Subsystem
  Constant{,1..5} (6 alike) : Constant  Value=0
  Multiport Switch1 : MultiPortSwitch  DataPortOrder=Zero-based contiguous  Inputs=5  zeroidx=on
  Saturation : Saturate  UpperLimit=1  LowerLimit=0
  Saturation1 : Saturate  UpperLimit=1.5  LowerLimit=0
  Switch{,1..3} (4 alike) : Switch  Criteria=u2 > Threshold
  alpha in engine start : Subsystem
  alphaBrTorque : Outport
  alphaTorque : Outport  Port=2
  wires:
  Constant2/1 -> Switch1/3
  Switch1/1 -> alphaTorque/1
  [EngStarted] -> Switch1/2
  Constant1/1 -> Switch/3
  Switch/1 -> alphaBrTorque/1
  [EngStarted] -> Switch/2
  Saturation/1 -> Switch/1
  Constant/1 -> Multiport Switch1/2
  AlphaFm calculation/1(alpha_fm) -> Saturation1/1
  mcm_trq_act_eff/1 -> AlphaFm calculation/1(mcm_trq_act_eff)
  AlphaBr3 calculation/1(alpha_br3) -> Multiport Switch1/5
  AlphaBr2 calculation/1(alpha_br2) -> Multiport Switch1/4
  AlphaBr1 calculation/1(alpha_br1) -> Multiport Switch1/3
  [brakingMode] -> Multiport Switch1/1
  mcm_act_braking_trq/1 -> AlphaBr3 calculation/1(mcm_act_braking_trq), AlphaBr2 calculation/1(mcm_act_braking_trq), AlphaBr1 calculation/1(mcm_act_braking_trq)
  [EngSpeed] -> AlphaBr1 calculation/2(EngSpeed), AlphaFm calculation/2(EngSpeed), alpha in engine start/3(EngSpeed), AlphaBr2 calculation/2(EngSpeed), AlphaBr3 calculation/2(EngSpeed)
  Multiport Switch1/1 -> Saturation/1
  Constant3/1 -> Multiport Switch1/6
  mcm_fbf_des_fuel_mass/1 -> Switch2/2
  Saturation1/1 -> Switch2/1
  Constant4/1 -> Switch2/3
  Constant5/1 -> Switch3/3
  mcm_EomEng_Stat_MCM/1 -> Switch3/2, alpha in engine start/2(mcm_EomEng_Stat_MCM)
  Switch2/1 -> Switch3/1
  Switch3/1 -> alpha in engine start/1(alpha_val)
  alpha in engine start/1(alphaTorque) -> Switch1/1

== system eng_simple_transient_std/eng_simple_transient_std/SetPoint_model/braking mode ==
  mcm_jb_active_bank1 : Inport
  mcm_jb_active_bank2 : Inport  Port=2
  mcm_tsa_itc_mode_act : Inport  Port=3
  Add : Sum  Inputs=+++
  Compare To Constant : simulink/Logic and Bit Operations/Compare To Constant  relop===  const=2  OutDataTypeStr=uint8
  Gain : Gain  Gain=2/100
  Gain1 : Gain  Gain=1/100
  Gain2 : Gain  Gain=4
  BrakingMode : Outport
  wires:
  mcm_jb_active_bank2/1 -> Gain/1
  Add/1 -> BrakingMode/1
  mcm_jb_active_bank1/1 -> Gain1/1
  Gain1/1 -> Add/1
  Gain/1 -> Add/2
  mcm_tsa_itc_mode_act/1 -> Compare To Constant/1
  Compare To Constant/1 -> Gain2/1
  Gain2/1 -> Add/3

== system eng_simple_transient_std/eng_simple_transient_std/Airpath_model/After air cooler calculation/T2N sensor filter ==
  T2N_flow_degC : Inport
  Constant : Constant
  Digital Clock : DigitalClock  SampleTime=-1
  Fcn : Fcn  Expr=u(2)/(u(2)+u(1))
  Initialisation : Switch  Criteria=u2 > Threshold
  Memory4 : Memory  InheritSampleTime=on
  Mux : Mux  Inputs=2
  Product : Product  SaturateOnIntegerOverflow=on  InputSameDT=on  OutDataTypeStr=Inherit: Same as first input
  Product1 : Product  SaturateOnIntegerOverflow=on  InputSameDT=on  OutDataTypeStr=Inherit: Same as first input
  Sum : Sum  Inputs=|+-  SaturateOnIntegerOverflow=on  InputSameDT=on  OutDataTypeStr=Inherit: Same as first input
  Sum1 : Sum  Inputs=|++  SaturateOnIntegerOverflow=on  InputSameDT=on  OutDataTypeStr=Inherit: Same as first input
  dt : Constant  Value=Fiter_calibration_dt
  tc T2N : Lookup  InputValues=Fiter_calibration_fmode_x_NMOT_rpm  Table=Fiter_calibration_fmode_y_tc_T2N  LookUpMeth=Interpolation-Use End Values
  T2N_degC : Outport
  wires:
  Initialisation/1 -> Memory4/1, T2N_degC/1
  Sum1/1 -> Initialisation/1
  Digital Clock/1 -> Initialisation/2
  [EngSpeed] -> tc T2N/1
  Fcn/1 -> Sum/2, Product1/1
  Constant/1 -> Sum/1
  Sum/1 -> Product/2
  Product1/1 -> Sum1/2
  Product/1 -> Sum1/1
  Memory4/1 -> Product/1
  T2N_flow_degC/1 -> Initialisation/3, Product1/2
  dt/1 -> Mux/2
  Mux/1 -> Fcn/1
  tc T2N/1 -> Mux/1

== system eng_simple_transient_std/eng_simple_transient_std/Airpath_model/After compressor calculation/T2V sensor filter ==
  T2V_flow_degC : Inport
  Constant : Constant
  Digital Clock : DigitalClock  SampleTime=-1
  Fcn : Fcn  Expr=u(2)/(u(2)+u(1))
  Initialisation : Switch  Criteria=u2 > Threshold
  Memory4 : Memory  InheritSampleTime=on
  Mux : Mux  Inputs=2
  Product : Product  SaturateOnIntegerOverflow=on  InputSameDT=on  OutDataTypeStr=Inherit: Same as first input
  Product1 : Product  SaturateOnIntegerOverflow=on  InputSameDT=on  OutDataTypeStr=Inherit: Same as first input
  Sum : Sum  Inputs=|+-  SaturateOnIntegerOverflow=on  InputSameDT=on  OutDataTypeStr=Inherit: Same as first input
  Sum1 : Sum  Inputs=|++  SaturateOnIntegerOverflow=on  InputSameDT=on  OutDataTypeStr=Inherit: Same as first input
  dt : Constant  Value=Fiter_calibration_dt
  tc T2V : Lookup  InputValues=Fiter_calibration_fmode_x_NMOT_rpm  Table=Fiter_calibration_fmode_y_tc_T2V  LookUpMeth=Interpolation-Use End Values
  T2V_degC : Outport
  wires:
  Initialisation/1 -> Memory4/1, T2V_degC/1
  Sum1/1 -> Initialisation/1
  Digital Clock/1 -> Initialisation/2
  tc T2V/1 -> Mux/1
  Mux/1 -> Fcn/1
  dt/1 -> Mux/2
  T2V_flow_degC/1 -> Initialisation/3, Product1/2
  Memory4/1 -> Product/1
  Product/1 -> Sum1/1
  Product1/1 -> Sum1/2
  Sum/1 -> Product/2
  Constant/1 -> Sum/1
  Fcn/1 -> Product1/1, Sum/2
  [EngSpeed] -> tc T2V/1

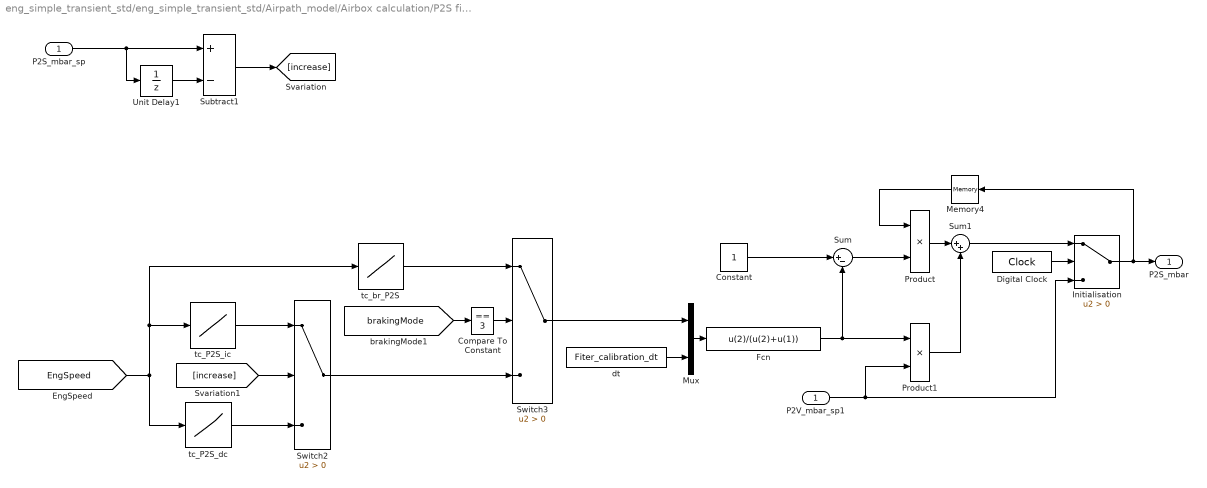
== system eng_simple_transient_std/eng_simple_transient_std/Airpath_model/Airbox calculation/P2S filter ==
  P2S_mbar_sp : Inport
  Compare To Constant : simulink/Logic and Bit Operations/Compare To Constant  relop===  const=3  OutDataTypeStr=uint8
  Constant : Constant
  Digital Clock : DigitalClock  SampleTime=-1
  Fcn : Fcn  Expr=u(2)/(u(2)+u(1))
  Initialisation : Switch  Criteria=u2 > Threshold
  Memory4 : Memory  InheritSampleTime=on
  Mux : Mux  Inputs=2
  P2V_mbar_sp1 : InportShadow
  Product : Product  SaturateOnIntegerOverflow=on  InputSameDT=on  OutDataTypeStr=Inherit: Same as first input
  Product1 : Product  SaturateOnIntegerOverflow=on  InputSameDT=on  OutDataTypeStr=Inherit: Same as first input
  Subtract1 : Sum  Inputs=+-
  Sum : Sum  Inputs=|+-  SaturateOnIntegerOverflow=on  InputSameDT=on  OutDataTypeStr=Inherit: Same as first input
  Sum1 : Sum  Inputs=|++  SaturateOnIntegerOverflow=on  InputSameDT=on  OutDataTypeStr=Inherit: Same as first input
  Switch2 : Switch  Criteria=u2 > Threshold
  Switch3 : Switch  Criteria=u2 > Threshold
  Unit Delay1 : UnitDelay  SampleTime=-1
  dt : Constant  Value=Fiter_calibration_dt
  tc_P2S_dc : Lookup  InputValues=Fiter_calibration_fmode_x_NMOT_rpm  Table=Fiter_calibration_fmode_y_tc_P2S_dc  LookUpMeth=Interpolation-Use End Values
  tc_P2S_ic : Lookup  InputValues=Fiter_calibration_fmode_x_NMOT_rpm  Table=Fiter_calibration_fmode_y_tc_P2S_ic  LookUpMeth=Interpolation-Use End Values
  tc_br_P2S : Lookup  InputValues=Fiter_calibration_brmode_x_NMOT_rpm  Table=Fiter_calibration_brmode_y_tc_P2S  LookUpMeth=Interpolation-Use End Values
  P2S_mbar : Outport
  wires:
  Initialisation/1 -> Memory4/1, P2S_mbar/1
  Sum1/1 -> Initialisation/1
  Digital Clock/1 -> Initialisation/2
  Product1/1 -> Sum1/2
  Product/1 -> Sum1/1
  Fcn/1 -> Sum/2, Product1/1
  Constant/1 -> Sum/1
  Sum/1 -> Product/2
  Memory4/1 -> Product/1
  P2V_mbar_sp1/1 -> Initialisation/3, Product1/2
  dt/1 -> Mux/2
  Switch3/1 -> Mux/1
  Mux/1 -> Fcn/1
  Unit Delay1/1 -> Subtract1/2
  Subtract1/1 -> [increase]
  P2S_mbar_sp/1 -> Subtract1/1, Unit Delay1/1
  [increase] -> Switch2/2
  [brakingMode] -> Compare To Constant/1
  Switch2/1 -> Switch3/3
  tc_br_P2S/1 -> Switch3/1
  [EngSpeed] -> tc_P2S_dc/1, tc_P2S_ic/1, tc_br_P2S/1
  tc_P2S_ic/1 -> Switch2/1
  tc_P2S_dc/1 -> Switch2/3
  Compare To Constant/1 -> Switch3/2

== system eng_simple_transient_std/eng_simple_transient_std/Airpath_model/Airbox calculation/T2S sensor filter ==
  T2S_flow_degC : Inport
  Constant : Constant
  Digital Clock : DigitalClock  SampleTime=-1
  Fcn : Fcn  Expr=u(2)/(u(2)+u(1))
  Initialisation : Switch  Criteria=u2 > Threshold
  Memory4 : Memory  InheritSampleTime=on
  Mux : Mux  Inputs=2
  Product : Product  SaturateOnIntegerOverflow=on  InputSameDT=on  OutDataTypeStr=Inherit: Same as first input
  Product1 : Product  SaturateOnIntegerOverflow=on  InputSameDT=on  OutDataTypeStr=Inherit: Same as first input
  Sum : Sum  Inputs=|+-  SaturateOnIntegerOverflow=on  InputSameDT=on  OutDataTypeStr=Inherit: Same as first input
  Sum1 : Sum  Inputs=|++  SaturateOnIntegerOverflow=on  InputSameDT=on  OutDataTypeStr=Inherit: Same as first input
  dt : Constant  Value=Fiter_calibration_dt
  tc T2V : Lookup  InputValues=Fiter_calibration_fmode_x_NMOT_rpm  Table=Fiter_calibration_fmode_y_tc_T2V  LookUpMeth=Interpolation-Use End Values
  T2S_degC : Outport
  wires:
  Initialisation/1 -> Memory4/1, T2S_degC/1
  Sum1/1 -> Initialisation/1
  Digital Clock/1 -> Initialisation/2
  [EngSpeed] -> tc T2V/1
  Fcn/1 -> Sum/2, Product1/1
  Constant/1 -> Sum/1
  Sum/1 -> Product/2
  Product1/1 -> Sum1/2
  Product/1 -> Sum1/1
  Memory4/1 -> Product/1
  T2S_flow_degC/1 -> Initialisation/3, Product1/2
  dt/1 -> Mux/2
  Mux/1 -> Fcn/1
  tc T2V/1 -> Mux/1

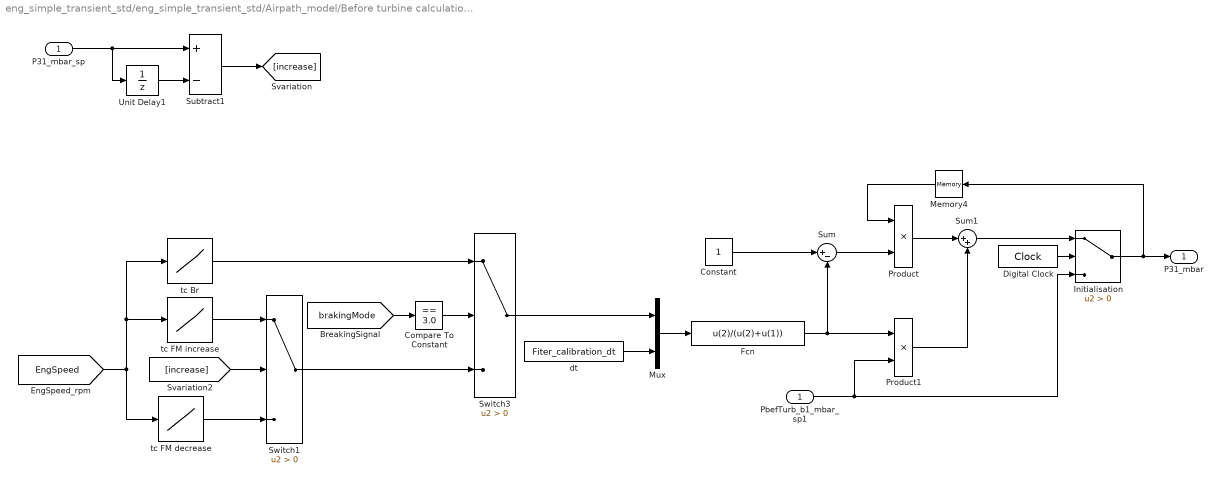
== system eng_simple_transient_std/eng_simple_transient_std/Airpath_model/Before turbine calculation/P31 filter ==
  P31_mbar_sp : Inport
  Compare To Constant : simulink/Logic and Bit Operations/Compare To Constant  relop===  const=3.0  OutDataTypeStr=uint8
  Constant : Constant
  Digital Clock : DigitalClock  SampleTime=-1
  Fcn : Fcn  Expr=u(2)/(u(2)+u(1))
  Initialisation : Switch  Criteria=u2 > Threshold
  Memory4 : Memory  InheritSampleTime=on
  Mux : Mux  Inputs=2
  PbefTurb_b1_mbar_sp1 : InportShadow
  Product : Product  SaturateOnIntegerOverflow=on  InputSameDT=on  OutDataTypeStr=Inherit: Same as first input
  Product1 : Product  SaturateOnIntegerOverflow=on  InputSameDT=on  OutDataTypeStr=Inherit: Same as first input
  Subtract1 : Sum  Inputs=+-
  Sum : Sum  Inputs=|+-  SaturateOnIntegerOverflow=on  InputSameDT=on  OutDataTypeStr=Inherit: Same as first input
  Sum1 : Sum  Inputs=|++  SaturateOnIntegerOverflow=on  InputSameDT=on  OutDataTypeStr=Inherit: Same as first input
  Switch1 : Switch  Criteria=u2 > Threshold
  Switch3 : Switch  Criteria=u2 > Threshold
  Unit Delay1 : UnitDelay  SampleTime=-1
  dt : Constant  Value=Fiter_calibration_dt
  tc Br : Lookup  InputValues=Fiter_calibration_brmode_x_NMOT_rpm  Table=Fiter_calibration_brmode_y_tc_P31  LookUpMeth=Interpolation-Use End Values
  tc FM decrease : Lookup  InputValues=Fiter_calibration_fmode_x_NMOT_rpm  Table=Fiter_calibration_fmode_y_tc_P31_dc  LookUpMeth=Interpolation-Use End Values
  tc FM increase : Lookup  InputValues=Fiter_calibration_fmode_x_NMOT_rpm  Table=Fiter_calibration_fmode_y_tc_P31_ic  LookUpMeth=Interpolation-Use End Values
  P31_mbar : Outport
  wires:
  Initialisation/1 -> Memory4/1, P31_mbar/1
  Sum1/1 -> Initialisation/1
  Digital Clock/1 -> Initialisation/2
  Switch3/1 -> Mux/1
  tc FM decrease/1 -> Switch1/3
  tc FM increase/1 -> Switch1/1
  [EngSpeed] -> tc Br/1, tc FM increase/1, tc FM decrease/1
  tc Br/1 -> Switch3/1
  Switch1/1 -> Switch3/3
  [brakingMode] -> Compare To Constant/1
  [increase] -> Switch1/2
  P31_mbar_sp/1 -> Unit Delay1/1, Subtract1/1
  Subtract1/1 -> [increase]
  Unit Delay1/1 -> Subtract1/2
  Mux/1 -> Fcn/1
  dt/1 -> Mux/2
  PbefTurb_b1_mbar_sp1/1 -> Initialisation/3, Product1/2
  Memory4/1 -> Product/1
  Product/1 -> Sum1/1
  Product1/1 -> Sum1/2
  Sum/1 -> Product/2
  Constant/1 -> Sum/1
  Fcn/1 -> Product1/1, Sum/2
  Compare To Constant/1 -> Switch3/2

== system eng_simple_transient_std/eng_simple_transient_std/Airpath_model/Before turbine calculation/P32 filter ==
  P32_mbar_sp : Inport
  Compare To Constant : simulink/Logic and Bit Operations/Compare To Constant  relop===  const=3.0  OutDataTypeStr=uint8
  Constant : Constant
  Digital Clock : DigitalClock  SampleTime=-1
  Fcn : Fcn  Expr=u(2)/(u(2)+u(1))
  Initialisation : Switch  Criteria=u2 > Threshold
  Memory4 : Memory  InheritSampleTime=on
  Mux : Mux  Inputs=2
  P32_mbar_sp1 : InportShadow
  Product : Product  SaturateOnIntegerOverflow=on  InputSameDT=on  OutDataTypeStr=Inherit: Same as first input
  Product1 : Product  SaturateOnIntegerOverflow=on  InputSameDT=on  OutDataTypeStr=Inherit: Same as first input
  Subtract1 : Sum  Inputs=+-
  Sum : Sum  Inputs=|+-  SaturateOnIntegerOverflow=on  InputSameDT=on  OutDataTypeStr=Inherit: Same as first input
  Sum1 : Sum  Inputs=|++  SaturateOnIntegerOverflow=on  InputSameDT=on  OutDataTypeStr=Inherit: Same as first input
  Switch1 : Switch  Criteria=u2 > Threshold
  Switch3 : Switch  Criteria=u2 > Threshold
  Unit Delay1 : UnitDelay  SampleTime=-1
  dt : Constant  Value=Fiter_calibration_dt
  tc Br : Lookup  InputValues=Fiter_calibration_brmode_x_NMOT_rpm  Table=Fiter_calibration_brmode_y_tc_P32  LookUpMeth=Interpolation-Use End Values
  tc FM decrease : Lookup  InputValues=Fiter_calibration_fmode_x_NMOT_rpm  Table=Fiter_calibration_fmode_y_tc_P32_dc  LookUpMeth=Interpolation-Use End Values
  tc FM increase : Lookup  InputValues=Fiter_calibration_fmode_x_NMOT_rpm  Table=Fiter_calibration_fmode_y_tc_P32_ic  LookUpMeth=Interpolation-Use End Values
  P32_mbar : Outport
  wires:
  Initialisation/1 -> Memory4/1, P32_mbar/1
  Sum1/1 -> Initialisation/1
  Digital Clock/1 -> Initialisation/2
  tc Br/1 -> Switch3/1
  Switch3/1 -> Mux/1
  tc FM decrease/1 -> Switch1/3
  tc FM increase/1 -> Switch1/1
  [EngSpeed] -> tc Br/1, tc FM increase/1, tc FM decrease/1
  Switch1/1 -> Switch3/3
  [brakingMode] -> Compare To Constant/1
  [increase] -> Switch1/2
  Fcn/1 -> Sum/2, Product1/1
  Constant/1 -> Sum/1
  Sum/1 -> Product/2
  Product1/1 -> Sum1/2
  Product/1 -> Sum1/1
  Memory4/1 -> Product/1
  P32_mbar_sp1/1 -> Initialisation/3, Product1/2
  dt/1 -> Mux/2
  Mux/1 -> Fcn/1
  Unit Delay1/1 -> Subtract1/2
  Subtract1/1 -> [increase]
  P32_mbar_sp/1 -> Subtract1/1, Unit Delay1/1
  Compare To Constant/1 -> Switch3/2

== system eng_simple_transient_std/eng_simple_transient_std/Airpath_model/Before turbine calculation/T31 filter ==
  T31_degC_sp : Inport
  Compare To Constant : simulink/Logic and Bit Operations/Compare To Constant  relop===  const=3.0  OutDataTypeStr=uint8
  Constant : Constant
  Digital Clock : DigitalClock  SampleTime=-1
  Fcn : Fcn  Expr=u(2)/(u(2)+u(1))
  Initialisation : Switch  Criteria=u2 > Threshold
  Memory4 : Memory  InheritSampleTime=on
  Mux : Mux  Inputs=2
  Product : Product  SaturateOnIntegerOverflow=on  InputSameDT=on  OutDataTypeStr=Inherit: Same as first input
  Product1 : Product  SaturateOnIntegerOverflow=on  InputSameDT=on  OutDataTypeStr=Inherit: Same as first input
  Subtract1 : Sum  Inputs=+-
  Sum : Sum  Inputs=|+-  SaturateOnIntegerOverflow=on  InputSameDT=on  OutDataTypeStr=Inherit: Same as first input
  Sum1 : Sum  Inputs=|++  SaturateOnIntegerOverflow=on  InputSameDT=on  OutDataTypeStr=Inherit: Same as first input
  Switch1 : Switch  Criteria=u2 > Threshold
  Switch3 : Switch  Criteria=u2 > Threshold
  T31_degC_sp1 : InportShadow
  Unit Delay1 : UnitDelay  SampleTime=-1
  dt : Constant  Value=Fiter_calibration_dt
  tc Br : Lookup  InputValues=Fiter_calibration_brmode_x_NMOT_rpm  Table=Fiter_calibration_brmode_y_tc_T31  LookUpMeth=Interpolation-Use End Values
  tc FM decrease : Lookup  InputValues=Fiter_calibration_fmode_x_NMOT_rpm  Table=Fiter_calibration_fmode_y_tc_T31_dc  LookUpMeth=Interpolation-Use End Values
  tc FM increase : Lookup  InputValues=Fiter_calibration_fmode_x_NMOT_rpm  Table=Fiter_calibration_fmode_y_tc_T31_ic  LookUpMeth=Interpolation-Use End Values
  T31_degC : Outport
  wires:
  Initialisation/1 -> Memory4/1, T31_degC/1
  Sum1/1 -> Initialisation/1
  Digital Clock/1 -> Initialisation/2
  Switch3/1 -> Mux/1
  tc FM decrease/1 -> Switch1/3
  tc FM increase/1 -> Switch1/1
  [EngSpeed] -> tc Br/1, tc FM increase/1, tc FM decrease/1
  tc Br/1 -> Switch3/1
  Switch1/1 -> Switch3/3
  [brakingMode] -> Compare To Constant/1
  [increase] -> Switch1/2
  Fcn/1 -> Sum/2, Product1/1
  Constant/1 -> Sum/1
  Sum/1 -> Product/2
  Product1/1 -> Sum1/2
  Product/1 -> Sum1/1
  Memory4/1 -> Product/1
  T31_degC_sp1/1 -> Initialisation/3, Product1/2
  dt/1 -> Mux/2
  Mux/1 -> Fcn/1
  Unit Delay1/1 -> Subtract1/2
  Subtract1/1 -> [increase]
  T31_degC_sp/1 -> Subtract1/1, Unit Delay1/1
  Compare To Constant/1 -> Switch3/2

== system eng_simple_transient_std/eng_simple_transient_std/Airpath_model/Before turbine calculation/T32 filter ==
  T32_degC_sp : Inport
  Compare To Constant : simulink/Logic and Bit Operations/Compare To Constant  relop===  const=3.0  OutDataTypeStr=uint8
  Constant : Constant
  Digital Clock : DigitalClock  SampleTime=-1
  Fcn : Fcn  Expr=u(2)/(u(2)+u(1))
  Initialisation : Switch  Criteria=u2 > Threshold
  Memory4 : Memory  InheritSampleTime=on
  Mux : Mux  Inputs=2
  Product : Product  SaturateOnIntegerOverflow=on  InputSameDT=on  OutDataTypeStr=Inherit: Same as first input
  Product1 : Product  SaturateOnIntegerOverflow=on  InputSameDT=on  OutDataTypeStr=Inherit: Same as first input
  Subtract1 : Sum  Inputs=+-
  Sum : Sum  Inputs=|+-  SaturateOnIntegerOverflow=on  InputSameDT=on  OutDataTypeStr=Inherit: Same as first input
  Sum1 : Sum  Inputs=|++  SaturateOnIntegerOverflow=on  InputSameDT=on  OutDataTypeStr=Inherit: Same as first input
  Switch1 : Switch  Criteria=u2 > Threshold
  Switch3 : Switch  Criteria=u2 > Threshold
  T32_degC_sp1 : InportShadow
  Unit Delay1 : UnitDelay  SampleTime=-1
  dt : Constant  Value=Fiter_calibration_dt
  tc Br : Lookup  InputValues=Fiter_calibration_brmode_x_NMOT_rpm  Table=Fiter_calibration_brmode_y_tc_T32  LookUpMeth=Interpolation-Use End Values
  tc FM decrease : Lookup  InputValues=Fiter_calibration_fmode_x_NMOT_rpm  Table=Fiter_calibration_fmode_y_tc_T32_dc  LookUpMeth=Interpolation-Use End Values
  tc FM increase : Lookup  InputValues=Fiter_calibration_fmode_x_NMOT_rpm  Table=Fiter_calibration_fmode_y_tc_T32_ic  LookUpMeth=Interpolation-Use End Values
  T32_degC : Outport
  wires:
  Initialisation/1 -> T32_degC/1, Memory4/1
  Sum1/1 -> Initialisation/1
  Digital Clock/1 -> Initialisation/2
  Switch3/1 -> Mux/1
  tc FM decrease/1 -> Switch1/3
  tc FM increase/1 -> Switch1/1
  [EngSpeed] -> tc Br/1, tc FM increase/1, tc FM decrease/1
  tc Br/1 -> Switch3/1
  Switch1/1 -> Switch3/3
  [brakingMode] -> Compare To Constant/1
  [increase] -> Switch1/2
  T32_degC_sp/1 -> Unit Delay1/1, Subtract1/1
  Subtract1/1 -> [increase]
  Unit Delay1/1 -> Subtract1/2
  Mux/1 -> Fcn/1
  dt/1 -> Mux/2
  T32_degC_sp1/1 -> Initialisation/3, Product1/2
  Memory4/1 -> Product/1
  Product/1 -> Sum1/1
  Product1/1 -> Sum1/2
  Sum/1 -> Product/2
  Constant/1 -> Sum/1
  Fcn/1 -> Product1/1, Sum/2
  Compare To Constant/1 -> Switch3/2
